simulink model "Modelo_Final"  (R2021a)
settings: Solver=VariableStepAuto  StartTime=0.0  StopTime=20  MaxStep=1e-5  RelTol=1e-3
values from neighbouring files (symbols this model uses):
  a1c = A1(2, 2)    [filtros_ss.m]
  a1m = a1c    [filtros_ss.m]
  a1p = A2(2, 2)    [filtros_ss.m]
  a1t = B3    [filtros_ss.m]
  a2c = A1(2, 1)    [filtros_ss.m]
  a2m = a2c    [filtros_ss.m]
  a2p = A2(2, 1)    [filtros_ss.m]
  a_cu = 3.9e-3    (= 0.0039)    [Datos.m]
  b_eq = 15.000e-6    (= 1.5e-05)    [Datos.m]
  ba = 0.0113    [Datos.m]
  Cts = 0.818    [Datos.m]
  Id_0 = 0    [Datos.m]
  J_eq = 5.6509e-6    (= 5.6509e-06)    [Datos.m]
  Ksa = 9.0414    [Datos.m]
  Ksia = 2893.2608    [Datos.m]
  lambda_m = 0.01546    [Datos.m]
  Ld = 6.6e-3    (= 0.0066)    [Datos.m]
  Lls = 0.8e-3    (= 0.0008)    [Datos.m]
  Lq = 5.8e-3    (= 0.0058)    [Datos.m]
  Pp = 3.01    [Datos.m]
  r = 314.3008    [Datos.m]
  Rs_ref = 1.02    [Datos.m]
  Rtsamb = 146.7    [Datos.m]
  sat = sqrt(2/3)*24    [filtros_ss.m]
  T_0 = 40.0    (= 40)    [Datos.m]
  T_amb = 40    [Datos.m]
  Tlmax = 6.28    [Datos.m]
  Ts_ref = 40    [Datos.m]
undefined symbols (not defined in the file or in its folder): mKi, mKtheta, mKw, R0, Rd, Rq
libraries: simulink x1
settings Model: Creator=ThnkPad  LastModifiedBy=jpss8

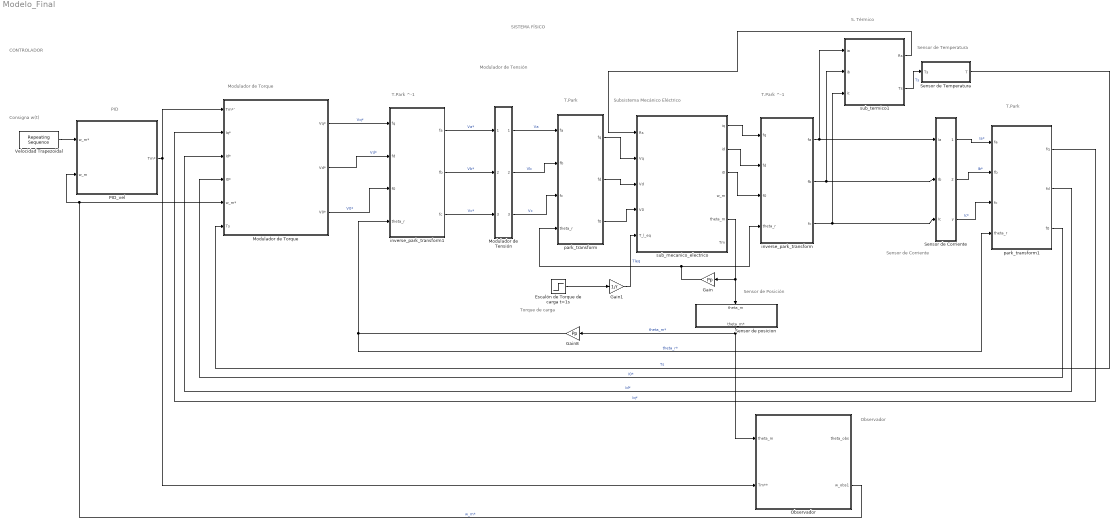
== system Modelo_Final ==
  note: Consigna w(t)
  note: CONTROLADOR
  note: SISTEMA FÍSICO
  note: PID
  note: Modulador de Torque
  note: T.Park ^-1
  note: Subsistema Mecánico Eléctrico
  note: S. Térmico
  note: T.Park ^-1
  note: T.Park
  note: Modulador
      | de
      | Tensión
  note: T.Park
  note: Observador
  note: Sensor de Posición
  note: Torque de carga
  note: Sensor de Corriente
  note: Sensor de Temperatura
  Escalón de Torque de carga t=1s : Step  After=Tlmax  SampleTime=0
  Gain : Gain  Gain=Pp
  Gain1 : Gain  Gain=1/r
  Gain8 : Gain  Gain=Pp
  Modulador de Tensión : Subsystem
  Modulador de Torque : Subsystem
  Observador : Subsystem
  PID_vel : Subsystem
  Sensor de Corriente : Subsystem
  Sensor de Temperatura : Subsystem
  Sensor de posicion : Subsystem
      settings: PortSchema="{\"entries\":[{\"content\":{\"sides\":[{\"content\":{\"connectorIds\":[]},\"type\":\"ConnectorPlacement.EquallySpacedRectSide\",\"uuid\":\"b536d0fd-a8b9-4fb9-bd2d-8cdbea63ffed\"},{\"content\":{\"connectorIds\":[],\"side\":\"RIGHT\"},\"type\":\"ConnectorPlacement.EquallySpacedRectSide\",\"uuid\":\"53663a0b-a681-499d-8c35-4379374d5e5a\"},{\"content\":{\"connectorIds\":[\"In1\"],\"side\":\"TOP\"},\"type\":\"ConnectorPlacement.EquallySpacedRectSide\",\"uuid\":\"1d4df5dd-d4dd-4e51-a644-5027fa847818\"},{\"content\":{\"connectorIds\":[\"Out1\"],\"side\":\"BOTTOM\"},\"type\":\"ConnectorPlacement.EquallySpacedRectSide\",\"uuid\":\"bae52777-b033-4852-a05b-da4dd91f0167\"}]},\"type\":\"ConnectorPlacement.EquallySpacedConnector\",\"uuid\":\"afdb905b-2ae6-4e5d-8f00-48d2cd8bae21\"}],\"packageUris\":[\"http://schema.mathworks.com/mf0/Connector/R2020b\"],\"version\":\"1.0\"}"
  Velocidad Trapezoidal : simulink/Sources/Repeating Sequence  rep_seq_t=t_sequence  rep_seq_y=w2
  inverse_park_transform : MATLAB Function  TreatAsAtomicUnit=on
  inverse_park_transform1 : MATLAB Function  TreatAsAtomicUnit=on
  park_transform : MATLAB Function  TreatAsAtomicUnit=on
  park_transform1 : MATLAB Function  TreatAsAtomicUnit=on
  sub_mecanico_electrico : Subsystem
  sub_termico1 : Subsystem
  wires:
  Sensor de Corriente/3(y) -> park_transform1/3(fc)  "Ic*"
  inverse_park_transform1/2(fb) -> Modulador de Tensión/2(Vb)  "Vb*"
  Modulador de Torque/2(Vd*) -> inverse_park_transform1/2(fd)  "Vd*"
  Sensor de Corriente/2(Out2) -> park_transform1/2(fb)  "Ib*"
  PID_vel/1(Tm*) -> Modulador de Torque/1(Tm*'), Observador/2(Tm**)
  park_transform1/3(f0) -> Modulador de Torque/4(I0*)  "I0*"
  park_transform1/1(fq) -> Modulador de Torque/2(Iq*)  "Iq*"
  inverse_park_transform1/1(fa) -> Modulador de Tensión/1(Va)  "Va*"
  Modulador de Torque/3(V0*) -> inverse_park_transform1/3(f0)  "V0*"
  Gain/1 -> park_transform/4(theta_r), inverse_park_transform/4(theta_r)
  sub_mecanico_electrico/5(theta_m) -> Sensor de posicion/1(theta_m), Gain/1
  inverse_park_transform1/3(fc) -> Modulador de Tensión/3(Vc)  "Vc*"
  inverse_park_transform/1(fa) -> sub_termico1/1(ia), Sensor de Corriente/1(Ia)
  inverse_park_transform/3(fc) -> sub_termico1/3(ic), Sensor de Corriente/3(Ic)
  park_transform/2(fd) -> sub_mecanico_electrico/3(Vd)
  sub_mecanico_electrico/1(iq) -> inverse_park_transform/1(fq)
  park_transform1/2(fd) -> Modulador de Torque/3(Id*)  "Id*"
  Gain8/1 -> park_transform1/4(theta_r), inverse_park_transform1/4(theta_r)  "theta_r*"
  park_transform/1(fq) -> sub_mecanico_electrico/2(Vq)
  park_transform/3(f0) -> sub_mecanico_electrico/4(V0)
  Sensor de posicion/1(theta_m*) -> Observador/1(theta_m), Gain8/1  "theta_m*"
  Modulador de Torque/1(Vq*) -> inverse_park_transform1/1(fq)  "Vq*"
  Modulador de Tensión/3(Vc*) -> park_transform/3(fc)  "Vc"
  Sensor de Corriente/1(Out1) -> park_transform1/1(fa)  "Ia*"
  inverse_park_transform/2(fb) -> sub_termico1/2(ib), Sensor de Corriente/2(Ib)
  Modulador de Tensión/1(Va*) -> park_transform/1(fa)  "Va"
  Observador/2(w_obs1) -> PID_vel/2(w_m), Modulador de Torque/5(w_m*)  "w_m*"
  Modulador de Tensión/2(Vb*) -> park_transform/2(fb)  "Vb"
  sub_mecanico_electrico/3(i0) -> inverse_park_transform/3(f0)
  Gain1/1 -> sub_mecanico_electrico/5(T_l_eq)  "Tleq"
  sub_mecanico_electrico/2(id) -> inverse_park_transform/2(fd)
  Velocidad Trapezoidal/1 -> PID_vel/1(w_m*)
  Escalón de Torque de carga t=1s/1 -> Gain1/1
  sub_termico1/2(Ts) -> Sensor de Temperatura/1(Ts)  "Ts"
  Sensor de Temperatura/1(T) -> Modulador de Torque/6(Ts)  "Ts"
  sub_termico1/1(Rs) -> sub_mecanico_electrico/1(Rs)

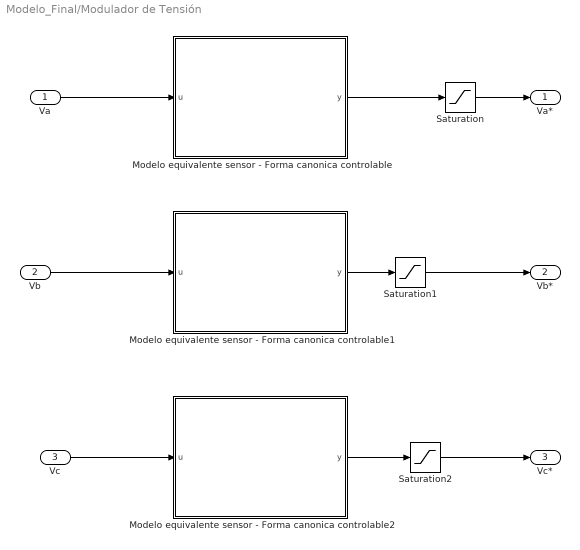
== system Modelo_Final/Modulador de Tensión ==
  Va : Inport
  Vb : Inport  Port=2
  Vc : Inport  Port=3
  Modelo equivalente sensor - Forma canonica controlable : Subsystem
  Modelo equivalente sensor - Forma canonica controlable1 : Subsystem
  Modelo equivalente sensor - Forma canonica controlable2 : Subsystem
  Saturation : Saturate  UpperLimit=sat  LowerLimit=-sat
  Saturation1 : Saturate  UpperLimit=sat  LowerLimit=-sat
  Saturation2 : Saturate  UpperLimit=sat  LowerLimit=-sat
  Va* : Outport
  Vb* : Outport  Port=2
  Vc* : Outport  Port=3
  wires:
  Va/1 -> Modelo equivalente sensor - Forma canonica controlable/1(u)
  Vb/1 -> Modelo equivalente sensor - Forma canonica controlable1/1(u)
  Vc/1 -> Modelo equivalente sensor - Forma canonica controlable2/1(u)
  Modelo equivalente sensor - Forma canonica controlable/1(y) -> Saturation/1
  Modelo equivalente sensor - Forma canonica controlable1/1(y) -> Saturation1/1
  Modelo equivalente sensor - Forma canonica controlable2/1(y) -> Saturation2/1
  Saturation1/1 -> Vb*/1
  Saturation2/1 -> Vc*/1
  Saturation/1 -> Va*/1

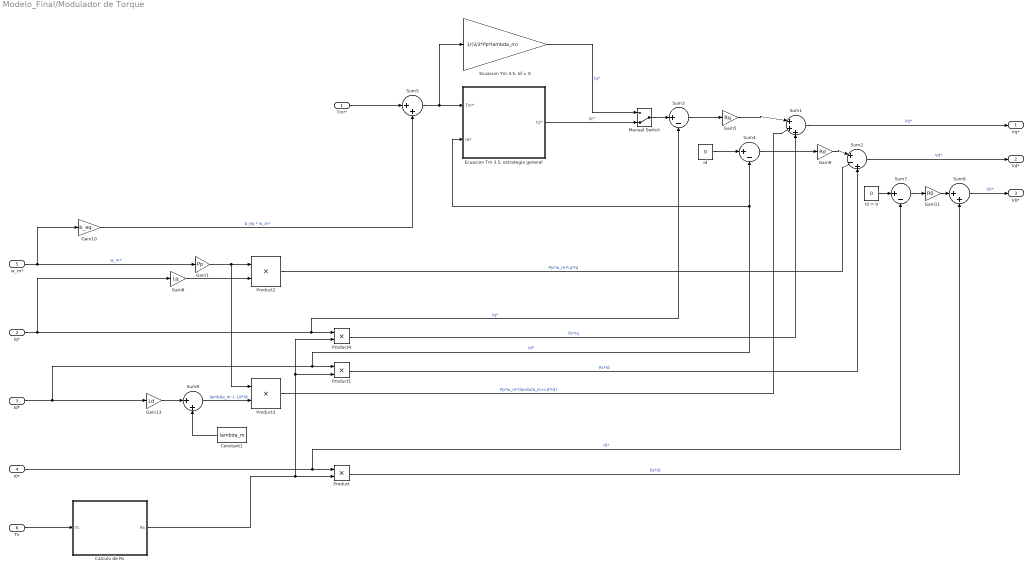
== system Modelo_Final/Modulador de Torque ==
  Tm*' : Inport
  Iq* : Inport  Port=2
  Id* : Inport  Port=3
  I0* : Inport  Port=4
  w_m* : Inport  Port=5
  Ts : Inport  Port=6
  Calculo de Rs : Subsystem
  Constant1 : Constant  Value=lambda_m
  "Ecuacion Tm 3.5, Id = 0" : Gain  Gain=1/(3/2*Pp*lambda_m)
  "Ecuacion Tm 3.5, estrategia general" : Subsystem
  Gain1 : Gain  Gain=Pp
  Gain10 : Gain  Gain=b_eq
  Gain11 : Gain  Gain=R0
  Gain13 : Gain  Gain=Ld
  Gain5 : Gain  Gain=Rq
  Gain8 : Gain  Gain=Lq
  Gain9 : Gain  Gain=Rd
  I0 = 0 : Constant  Value=0
  Id : Constant  Value=0
  Manual Switch : ManualSwitch  CurrentSetting=0
  Product{,1..4} (5 alike) : Product
  Sum1 : Sum  Inputs=|+++
  Sum2 : Sum  Inputs=|+-+
  Sum3 : Sum  Inputs=|+-
  Sum4 : Sum  Inputs=|+-
  Sum5 : Sum  Inputs=|++
  Sum6 : Sum  Inputs=|++
  Sum7 : Sum  Inputs=|+-
  Sum8 : Sum  Inputs=|++
  Vq* : Outport
  Vd* : Outport  Port=2
  V0* : Outport  Port=3
  wires:
  Sum7/1 -> Gain11/1
  I0 = 0/1 -> Sum7/1
  Tm*'/1 -> Sum5/1
  "Ecuacion Tm 3.5, Id = 0"/1 -> Manual Switch/1  "Iq*"
  Sum4/1 -> Gain9/1
  Sum5/1 -> "Ecuacion Tm 3.5, Id = 0"/1, "Ecuacion Tm 3.5, estrategia general"/1(Tm*')
  Id/1 -> Sum4/1
  Gain5/1 -> Sum1/1
  Gain9/1 -> Sum2/1
  Sum3/1 -> Gain5/1
  Sum2/1 -> Vd*/1  "Vd*"
  Gain11/1 -> Sum6/1
  Sum1/1 -> Vq*/1  "Vq*"
  Gain10/1 -> Sum5/2  "b_eq * w_m*"
  Product4/1 -> Sum1/3  "Rs*Iq"
  Product2/1 -> Sum2/2  "-Pp*w_m*Lq*Iq"
  Product1/1 -> Sum2/3  "Rs*Id"
  Product/1 -> Sum6/2  "Rs*I0"
  Product3/1 -> Sum1/2  "Pp*w_m*(lambda_m+Ld*Id)"
  w_m*/1 -> Gain10/1, Gain1/1  "w_m*"
  Iq*/1 -> Product4/1, Sum3/2, Gain8/1  "Iq*"
  Gain13/1 -> Sum8/1
  Gain8/1 -> Product2/2
  Gain1/1 -> Product3/1, Product2/1
  Constant1/1 -> Sum8/2
  Sum8/1 -> Product3/2  "lambda_m + Ld*Id"
  Id*/1 -> Product1/1, "Ecuacion Tm 3.5, estrategia general"/2(Id*), Sum4/2, Gain13/1  "Id*"
  I0*/1 -> Product/1, Sum7/2  "I0*"
  Sum6/1 -> V0*/1  "V0*"
  "Ecuacion Tm 3.5, estrategia general"/1(Iq*') -> Manual Switch/2  "Iq*'"
  Manual Switch/1 -> Sum3/1
  Ts/1 -> Calculo de Rs/1(Ts)
  Calculo de Rs/1(Rs) -> Product1/2, Product4/2, Product/2

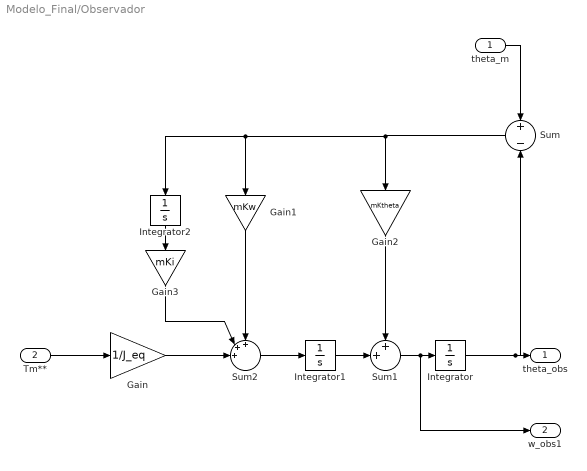
== system Modelo_Final/Observador ==
  theta_m : Inport
  Tm** : Inport  Port=2
  Gain : Gain  Gain=1/J_eq
  Gain1 : Gain  Gain=mKw
  Gain2 : Gain  Gain=mKtheta
  Gain3 : Gain  Gain=mKi
  Integrator : Integrator
  Integrator1 : Integrator
  Integrator2 : Integrator
  Sum : Sum  Inputs=+|-
  Sum1 : Sum  Inputs=++|
  Sum2 : Sum  Inputs=+++||
  theta_obs : Outport
  w_obs1 : Outport  Port=2
  wires:
  Integrator/1 -> Sum/2, theta_obs/1
  Sum2/1 -> Integrator1/1
  Sum/1 -> Integrator2/1, Gain1/1, Gain2/1
  theta_m/1 -> Sum/1
  Tm**/1 -> Gain/1
  Gain1/1 -> Sum2/1
  Gain2/1 -> Sum1/1
  Integrator1/1 -> Sum1/2
  Sum1/1 -> w_obs1/1, Integrator/1
  Gain/1 -> Sum2/3
  Gain3/1 -> Sum2/2
  Integrator2/1 -> Gain3/1

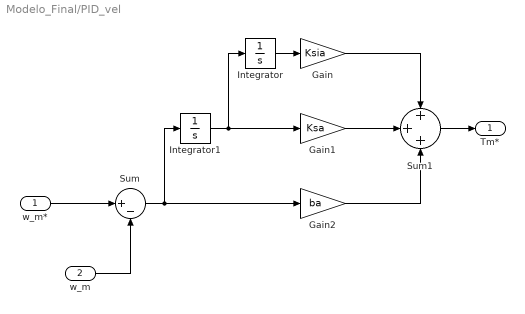
== system Modelo_Final/PID_vel ==
  w_m* : Inport
  w_m : Inport  Port=2
  Gain : Gain  Gain=Ksia
  Gain1 : Gain  Gain=Ksa
  Gain2 : Gain  Gain=ba
  Integrator : Integrator
  Integrator1 : Integrator
  Sum : Sum  Inputs=|+-
  Sum1 : Sum  Inputs=+++
  Tm* : Outport
  wires:
  Gain1/1 -> Sum1/2
  Sum1/1 -> Tm*/1
  Sum/1 -> Integrator1/1, Gain2/1
  Integrator/1 -> Gain/1
  Gain2/1 -> Sum1/3
  Gain/1 -> Sum1/1
  Integrator1/1 -> Gain1/1, Integrator/1
  w_m*/1 -> Sum/1
  w_m/1 -> Sum/2

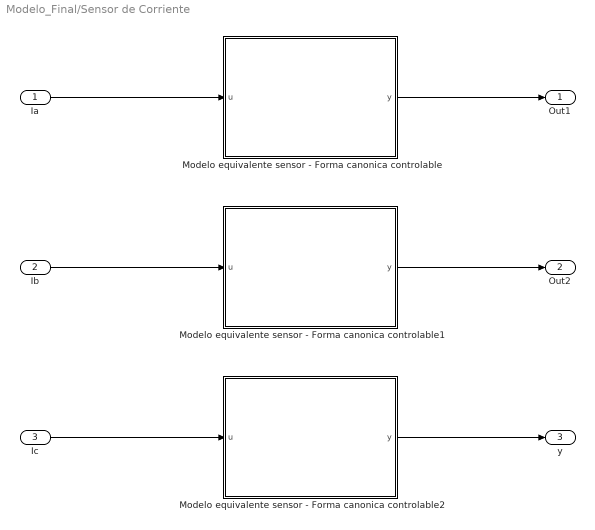
== system Modelo_Final/Sensor de Corriente ==
  Ia : Inport
  Ib : Inport  Port=2
  Ic : Inport  Port=3
  Modelo equivalente sensor - Forma canonica controlable : Subsystem
  Modelo equivalente sensor - Forma canonica controlable1 : Subsystem
  Modelo equivalente sensor - Forma canonica controlable2 : Subsystem
  Out1 : Outport
  Out2 : Outport  Port=2
  y : Outport  Port=3
  wires:
  Ic/1 -> Modelo equivalente sensor - Forma canonica controlable2/1(u)
  Ib/1 -> Modelo equivalente sensor - Forma canonica controlable1/1(u)
  Ia/1 -> Modelo equivalente sensor - Forma canonica controlable/1(u)
  Modelo equivalente sensor - Forma canonica controlable1/1(y) -> Out2/1
  Modelo equivalente sensor - Forma canonica controlable/1(y) -> Out1/1
  Modelo equivalente sensor - Forma canonica controlable2/1(y) -> y/1

== system Modelo_Final/Sensor de Temperatura ==
  Ts : Inport
  Gain : Gain
  Manual Switch : ManualSwitch
  Modelo equivalente sensor - Forma canonica controlable : Subsystem
  T : Outport
  wires:
  Ts/1 -> Modelo equivalente sensor - Forma canonica controlable/1(u), Gain/1
  Modelo equivalente sensor - Forma canonica controlable/1(y) -> Manual Switch/1
  Manual Switch/1 -> T/1
  Gain/1 -> Manual Switch/2

== system Modelo_Final/Sensor de posicion ==
  theta_m : Inport
  Modelo equivalente sensor - Forma canonica controlable : Subsystem
  theta_m* : Outport
  wires:
  theta_m/1 -> Modelo equivalente sensor - Forma canonica controlable/1(u)
  Modelo equivalente sensor - Forma canonica controlable/1(y) -> theta_m*/1

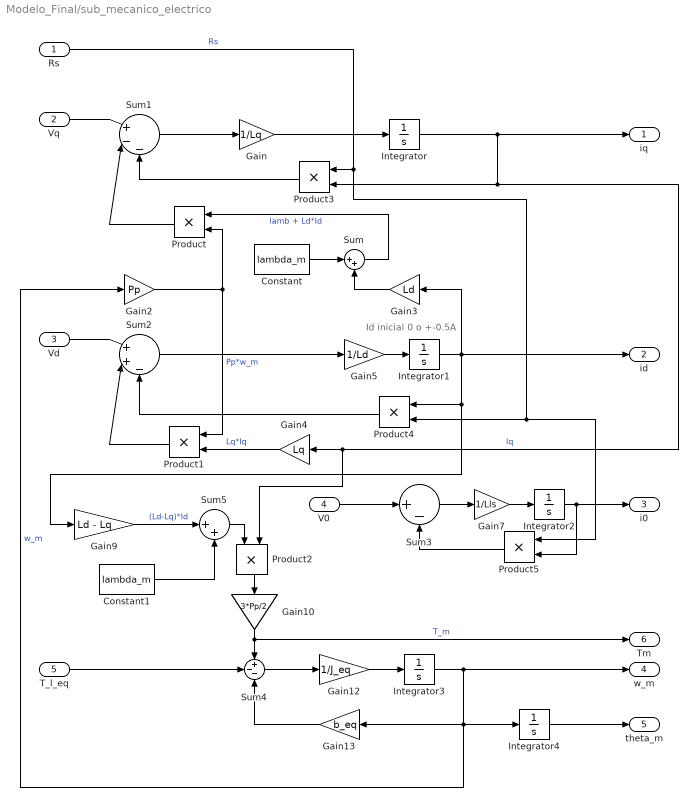
== system Modelo_Final/sub_mecanico_electrico ==
  note: Id inicial 0 o +-0.5A
  Rs : Inport
  Vq : Inport  Port=2
  Vd : Inport  Port=3
  V0 : Inport  Port=4
  T_l_eq : Inport  Port=5
  Constant : Constant  Value=lambda_m
  Constant1 : Constant  Value=lambda_m
  Gain : Gain  Gain=1/Lq
  Gain10 : Gain  Gain=3*Pp/2
  Gain12 : Gain  Gain=1/J_eq
  Gain13 : Gain  Gain=b_eq
  Gain2 : Gain  Gain=Pp
  Gain3 : Gain  Gain=Ld
  Gain4 : Gain  Gain=Lq
  Gain5 : Gain  Gain=1/Ld
  Gain7 : Gain  Gain=1/Lls
  Gain9 : Gain  Gain=Ld - Lq
  Integrator{,2..4} (4 alike) : Integrator
  Integrator1 : Integrator  InitialCondition=Id_0
  Product{,1..5} (6 alike) : Product
  Sum : Sum  Inputs=|++
  Sum1 : Sum  Inputs=|+--
  Sum2 : Sum  Inputs=|++-
  Sum3 : Sum  Inputs=|+-
  Sum4 : Sum  Inputs=+--
  Sum5 : Sum  Inputs=|++
  iq : Outport
  id : Outport  Port=2
  i0 : Outport  Port=3
  w_m : Outport  Port=4
  theta_m : Outport  Port=5
  Tm : Outport  Port=6
  wires:
  Gain12/1 -> Integrator3/1
  T_l_eq/1 -> Sum4/2
  Sum4/1 -> Gain12/1
  Gain10/1 -> Tm/1, Sum4/1  "T_m"
  Integrator4/1 -> theta_m/1
  Gain13/1 -> Sum4/3
  Integrator3/1 -> Gain2/1, Integrator4/1, Gain13/1, w_m/1  "w_m"
  Constant1/1 -> Sum5/2
  Gain9/1 -> Sum5/1  "(Ld-Lq)*Id"
  Sum5/1 -> Product2/1
  Product2/1 -> Gain10/1
  V0/1 -> Sum3/1
  Product5/1 -> Sum3/2
  Gain5/1 -> Integrator1/1
  Sum2/1 -> Gain5/1
  Integrator1/1 -> Product4/1, Gain9/1, id/1, Gain3/1
  Product/1 -> Sum1/2
  Integrator2/1 -> Product5/2, i0/1
  Product1/1 -> Sum2/2
  Gain4/1 -> Product1/2  "Lq*Iq"
  Product3/1 -> Sum1/3
  Product4/1 -> Sum2/3
  Sum/1 -> Product/1  "lamb + Ld*Id"
  Sum3/1 -> Gain7/1
  Gain7/1 -> Integrator2/1
  Vd/1 -> Sum2/1
  Gain3/1 -> Sum/2
  Gain2/1 -> Product1/1, Product/2  "Pp*w_m"
  Integrator/1 -> Product3/2, Gain4/1, Product2/2, iq/1  "Iq"
  Sum1/1 -> Gain/1
  Gain/1 -> Integrator/1
  Constant/1 -> Sum/1
  Vq/1 -> Sum1/1
  Rs/1 -> Product5/1, Product4/2, Product3/1  "Rs"

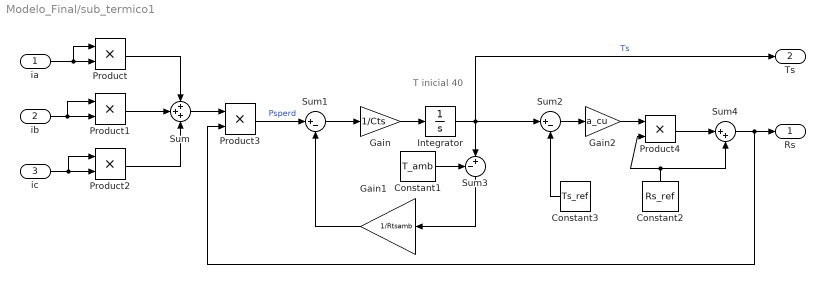
== system Modelo_Final/sub_termico1 ==
  note: T inicial 40
  ia : Inport
  ib : Inport  Port=2
  ic : Inport  Port=3
  Constant1 : Constant  Value=T_amb
  Constant2 : Constant  Value=Rs_ref
  Constant3 : Constant  Value=Ts_ref
  Gain : Gain  Gain=1/Cts
  Gain1 : Gain  Gain=1/Rtsamb
  Gain2 : Gain  Gain=a_cu
  Integrator : Integrator  InitialCondition=T_0
  Product{,1..4} (5 alike) : Product
  Sum : Sum  Inputs=+++
  Sum1 : Sum  Inputs=|+-
  Sum2 : Sum  Inputs=|+-
  Sum3 : Sum  Inputs=-+|
  Sum4 : Sum  Inputs=|++
  Rs : Outport
  Ts : Outport  Port=2
  wires:
  ic/1 -> Product2/1, Product2/2
  ib/1 -> Product1/1, Product1/2
  ia/1 -> Product/1, Product/2
  Product/1 -> Sum/1
  Product1/1 -> Sum/2
  Product2/1 -> Sum/3
  Product3/1 -> Sum1/1  "Psperd"
  Sum/1 -> Product3/1
  Sum4/1 -> Rs/1, Product3/2
  Gain1/1 -> Sum1/2
  Gain/1 -> Integrator/1
  Sum1/1 -> Gain/1
  Integrator/1 -> Ts/1, Sum2/1, Sum3/2  "Ts"
  Sum3/1 -> Gain1/1
  Constant1/1 -> Sum3/1
  Sum2/1 -> Gain2/1
  Gain2/1 -> Product4/1
  Product4/1 -> Sum4/1
  Constant2/1 -> Product4/2, Sum4/2
  Constant3/1 -> Sum2/2

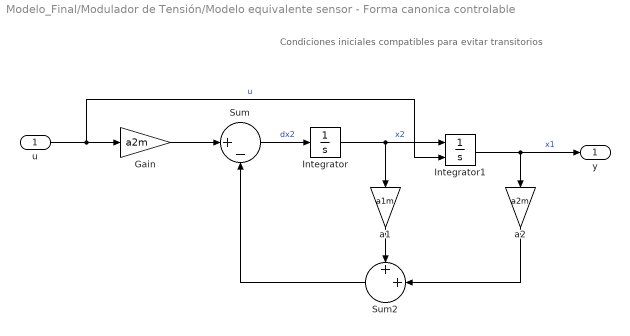
== system Modelo_Final/Modulador de Tensión/Modelo equivalente sensor - Forma canonica controlable ==
  note: Condiciones iniciales compatibles para evitar transitorios
  u : Inport
  Gain : Gain  Gain=a2m
  Integrator : Integrator
  Integrator1 : Integrator  InitialConditionSource=external
  Sum : Sum  Inputs=|+-
  Sum2 : Sum  Inputs=++|
  a1 : Gain  Gain=a1m
  a2 : Gain  Gain=a2m
  y : Outport
  wires:
  Sum/1 -> Integrator/1  "dx2"
  Integrator/1 -> a1/1, Integrator1/1  "x2"
  a1/1 -> Sum2/1
  Integrator1/1 -> y/1, a2/1  "x1"
  a2/1 -> Sum2/2
  Sum2/1 -> Sum/2
  u/1 -> Integrator1/2, Gain/1  "u"
  Gain/1 -> Sum/1

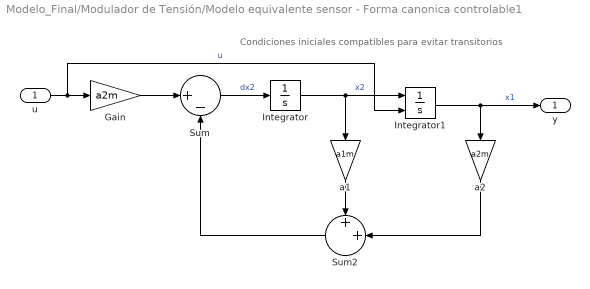
== system Modelo_Final/Modulador de Tensión/Modelo equivalente sensor - Forma canonica controlable1 ==
  note: Condiciones iniciales compatibles para evitar transitorios
  u : Inport
  Gain : Gain  Gain=a2m
  Integrator : Integrator
  Integrator1 : Integrator  InitialConditionSource=external
  Sum : Sum  Inputs=|+-
  Sum2 : Sum  Inputs=++|
  a1 : Gain  Gain=a1m
  a2 : Gain  Gain=a2m
  y : Outport
  wires:
  Sum/1 -> Integrator/1  "dx2"
  Integrator/1 -> a1/1, Integrator1/1  "x2"
  a1/1 -> Sum2/1
  Integrator1/1 -> y/1, a2/1  "x1"
  a2/1 -> Sum2/2
  Sum2/1 -> Sum/2
  u/1 -> Integrator1/2, Gain/1  "u"
  Gain/1 -> Sum/1

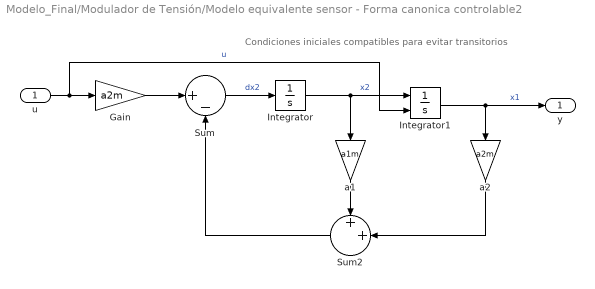
== system Modelo_Final/Modulador de Tensión/Modelo equivalente sensor - Forma canonica controlable2 ==
  note: Condiciones iniciales compatibles para evitar transitorios
  u : Inport
  Gain : Gain  Gain=a2m
  Integrator : Integrator
  Integrator1 : Integrator  InitialConditionSource=external
  Sum : Sum  Inputs=|+-
  Sum2 : Sum  Inputs=++|
  a1 : Gain  Gain=a1m
  a2 : Gain  Gain=a2m
  y : Outport
  wires:
  Sum/1 -> Integrator/1  "dx2"
  Integrator/1 -> a1/1, Integrator1/1  "x2"
  a1/1 -> Sum2/1
  Integrator1/1 -> y/1, a2/1  "x1"
  a2/1 -> Sum2/2
  Sum2/1 -> Sum/2
  u/1 -> Integrator1/2, Gain/1  "u"
  Gain/1 -> Sum/1

== system Modelo_Final/Modulador de Torque/Calculo de Rs ==
  Ts : Inport
  Constant2 : Constant  Value=Rs_ref
  Constant3 : Constant  Value=Ts_ref
  Gain2 : Gain  Gain=a_cu
  Product4 : Product
  Sum2 : Sum  Inputs=|+-
  Sum4 : Sum  Inputs=|++
  Rs : Outport
  wires:
  Gain2/1 -> Product4/1
  Constant3/1 -> Sum2/2
  Product4/1 -> Sum4/1
  Sum2/1 -> Gain2/1
  Ts/1 -> Sum2/1  "Ts"
  Constant2/1 -> Product4/2, Sum4/2
  Sum4/1 -> Rs/1

== system Modelo_Final/Modulador de Torque/Ecuacion Tm 3.5, estrategia general ==
  Tm*' : Inport
  Id* : Inport  Port=2
  Constant : Constant  Value=lambda_m
  Divide : Product  Inputs=*/
  Gain : Gain  Gain=3/2 * Pp
  Gain1 : Gain  Gain=Ld-Lq
  Sum : Sum  Inputs=|++
  Iq*' : Outport
  wires:
  Tm*'/1 -> Divide/1
  Id*/1 -> Gain1/1
  Gain1/1 -> Sum/1
  Constant/1 -> Sum/2
  Sum/1 -> Gain/1
  Divide/1 -> Iq*'/1
  Gain/1 -> Divide/2

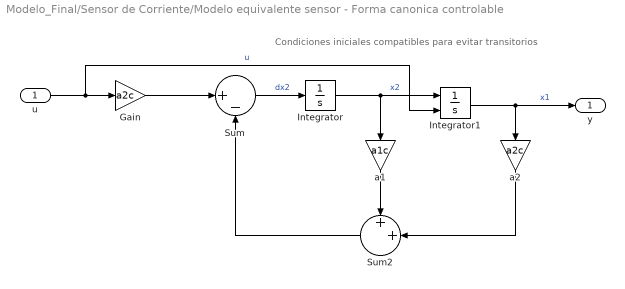
== system Modelo_Final/Sensor de Corriente/Modelo equivalente sensor - Forma canonica controlable ==
  note: Condiciones iniciales compatibles para evitar transitorios
  u : Inport
  Gain : Gain  Gain=a2c
  Integrator : Integrator
  Integrator1 : Integrator  InitialConditionSource=external
  Sum : Sum  Inputs=|+-
  Sum2 : Sum  Inputs=++|
  a1 : Gain  Gain=a1c
  a2 : Gain  Gain=a2c
  y : Outport
  wires:
  u/1 -> Integrator1/2, Gain/1  "u"
  Sum/1 -> Integrator/1  "dx2"
  Integrator/1 -> a1/1, Integrator1/1  "x2"
  a1/1 -> Sum2/1
  Integrator1/1 -> y/1, a2/1  "x1"
  a2/1 -> Sum2/2
  Sum2/1 -> Sum/2
  Gain/1 -> Sum/1

== system Modelo_Final/Sensor de Corriente/Modelo equivalente sensor - Forma canonica controlable1 ==
  note: Condiciones iniciales compatibles para evitar transitorios
  u : Inport
  Gain : Gain  Gain=a2c
  Integrator : Integrator
  Integrator1 : Integrator  InitialConditionSource=external
  Sum : Sum  Inputs=|+-
  Sum2 : Sum  Inputs=++|
  a1 : Gain  Gain=a1c
  a2 : Gain  Gain=a2c
  y : Outport
  wires:
  u/1 -> Integrator1/2, Gain/1  "u"
  Sum/1 -> Integrator/1  "dx2"
  Integrator/1 -> a1/1, Integrator1/1  "x2"
  a1/1 -> Sum2/1
  Integrator1/1 -> y/1, a2/1  "x1"
  a2/1 -> Sum2/2
  Sum2/1 -> Sum/2
  Gain/1 -> Sum/1

== system Modelo_Final/Sensor de Corriente/Modelo equivalente sensor - Forma canonica controlable2 ==
  note: Condiciones iniciales compatibles para evitar transitorios
  u : Inport
  Gain : Gain  Gain=a2c
  Integrator : Integrator
  Integrator1 : Integrator  InitialConditionSource=external
  Sum : Sum  Inputs=|+-
  Sum2 : Sum  Inputs=++|
  a1 : Gain  Gain=a1c
  a2 : Gain  Gain=a2c
  y : Outport
  wires:
  Sum/1 -> Integrator/1  "dx2"
  Integrator/1 -> a1/1, Integrator1/1  "x2"
  a1/1 -> Sum2/1
  Integrator1/1 -> y/1, a2/1  "x1"
  a2/1 -> Sum2/2
  Sum2/1 -> Sum/2
  u/1 -> Integrator1/2, Gain/1  "u"
  Gain/1 -> Sum/1

== system Modelo_Final/Sensor de Temperatura/Modelo equivalente sensor - Forma canonica controlable ==
  note: Condiciones iniciales compatibles para evitar transitorios
  u : Inport
  Integrator : Integrator  InitialConditionSource=external  InitialCondition=T_0
  Sum : Sum  Inputs=|+-
  a1 : Gain  Gain=a1t
  a1. : Gain  Gain=a1t
  y : Outport
  wires:
  u/1 -> Integrator/2, a1./1  "u"
  Sum/1 -> Integrator/1  "dx1"
  Integrator/1 -> y/1, a1/1  "x1"
  a1/1 -> Sum/2
  a1./1 -> Sum/1

== system Modelo_Final/Sensor de posicion/Modelo equivalente sensor - Forma canonica controlable ==
  note: Condiciones iniciales compatibles para evitar transitorios
  u : Inport
  Gain : Gain  Gain=a2p
  Integrator : Integrator
  Integrator1 : Integrator  InitialConditionSource=external
  Sum : Sum  Inputs=|+-
  Sum2 : Sum  Inputs=++|
  a1 : Gain  Gain=a1p
  a2 : Gain  Gain=a2p
  y : Outport
  wires:
  u/1 -> Integrator1/2, Gain/1  "u"
  Sum/1 -> Integrator/1  "dx2"
  Integrator/1 -> a1/1, Integrator1/1  "x2"
  a1/1 -> Sum2/1
  Integrator1/1 -> y/1, a2/1  "x1"
  a2/1 -> Sum2/2
  Sum2/1 -> Sum/2
  Gain/1 -> Sum/1

== matlab function Modelo_Final/inverse_park_transform ==
  data: fq input; fa output; fd input; f0 input; theta_r input; fb output; fc output
function [fa, fb, fc] =  inverse_park_transform(fq, fd, f0, theta_r)

ITP = [cos(theta_r)             sin(theta_r)           1;
       cos(theta_r - 2*pi/3)    sin(theta_r - 2*pi/3)  1;
       cos(theta_r + 2*pi/3)    sin(theta_r + 2*pi/3)  1];

abc = ITP*[fq; fd; f0];

fa = abc(1);
fb = abc(2);
fc = abc(3);
end

== matlab function Modelo_Final/inverse_park_transform1 ==
  data: fq input; fa output; fd input; f0 input; theta_r input; fb output; fc output
function [fa, fb, fc] =  inverse_park_transform(fq, fd, f0, theta_r)

ITP = [cos(theta_r)             sin(theta_r)           1;
       cos(theta_r - 2*pi/3)    sin(theta_r - 2*pi/3)  1;
       cos(theta_r + 2*pi/3)    sin(theta_r + 2*pi/3)  1];

abc = ITP*[fq; fd; f0];

fa = abc(1);
fb = abc(2);
fc = abc(3);
end

== matlab function Modelo_Final/park_transform ==
  data: fa input; fq output; fb input; fc input; theta_r input; fd output; f0 output
function [fq, fd, f0] =  park_transform(fa, fb, fc, theta_r)
    
TP = 2/3*[cos(theta_r)  cos(theta_r - 2*pi/3)   cos(theta_r + 2*pi/3);
          sin(theta_r)  sin(theta_r - 2*pi/3)   sin(theta_r + 2*pi/3);
          1/2           1/2                     1/2];
     
qd0 = TP*[fa; fb; fc];

fq = qd0(1);
fd = qd0(2);
f0 = qd0(3);
end

== matlab function Modelo_Final/park_transform1 ==
  data: fa input; fq output; fb input; fc input; theta_r input; fd output; f0 output
function [fq, fd, f0] =  park_transform(fa, fb, fc, theta_r)
    
TP = 2/3*[cos(theta_r)  cos(theta_r - 2*pi/3)   cos(theta_r + 2*pi/3);
          sin(theta_r)  sin(theta_r - 2*pi/3)   sin(theta_r + 2*pi/3);
          1/2           1/2                     1/2];
     
qd0 = TP*[fa; fb; fc];

fq = qd0(1);
fd = qd0(2);
f0 = qd0(3);
end
